simulink model "simulink_discrete1Dy3D_MatLab_function_mascara"  (R2023b)
settings: Solver=ode45  StartTime=0.0  StopTime=0.7  RelTol=1e-3  EnableMultiTasking=on
values from neighbouring files (symbols this model uses):
  a1 = C_discrete.den{1,1}(2)    [control_float_test.m]
  a2 = C_discrete.den{1,1}(3)    [control_float_test.m]
  b0 = C_discrete.num{1,1}(1)    [control_float_test.m]
  b1 = C_discrete.num{1,1}(2)    [control_float_test.m]
  b2 = C_discrete.num{1,1}(3)    [control_float_test.m]
  T = T2    (= 0.001)    [control_float_test.m]
libraries: cstblocks x4
settings Model: Creator=Koldo  LastModifiedBy=chris
settings SolverCC: AlgebraicLoopSolver=TrustRegion
settings DataIOCC: LimitDataPoints=on  SaveFormat=Array  SignalLoggingSaveFormat=ModelDataLogs  ReturnWorkspaceOutputs=off
settings OptimizationCC: ExpressionDepthLimit=2147483647  LifeSpan=inf
settings DebuggingCC: UnderspecifiedInitializationDetection=Classic  MergeDetectMultiDrivingBlocksExec=none  SolverPrmCheckMsg=warning  FcnCallInpInsideContextMsg=warning  UnconnectedInputMsg=warning  UnconnectedOutputMsg=warning  UnconnectedLineMsg=warning  StateNameClashWarn=warning  SFUnexpectedBacktrackingDiag=warning  SFNoUnconditionalDefaultTransitionDiag=warning  SFExecutionAtInitializationDiag=none  ArithmeticOperatorsInVariantConditions=warning
settings HardwareCC: ProdBitPerPointer=32  ProdBitPerSizeT=32  ProdBitPerPtrDiffT=32  ProdLargestAtomicFloat=None  ProdIntDivRoundTo=Undefined  ProdEndianess=Unspecified  ProdWordSize=32  ProdHWDeviceType=32-bit Generic
settings ModelReferenceCC: EnableRefExpFcnMdlSchedulingChecks=on  PropagateSignalLabelsOutOfModel=off
settings SFSimCC: SimUseLocalCustomCode=off  CustomCodeUndefinedFunction=UseInterfaceOnly
settings RTWCC: RTWUseLocalCustomCode=off  DLArmComputeVersion=19.05
settings CodeAppCC: StateflowObjectComments=on
settings GRTTargetCC: TargetLangStandard=C89/C90 (ANSI)  CombineOutputUpdateFcns=off  GRTInterface=on
settings ConfigComp: CovMetricSettings=dw  CovSaveCumulativeToWorkspaceVar=on  CovSaveSingleToWorkspaceVar=on  CovExternalEMLEnable=off

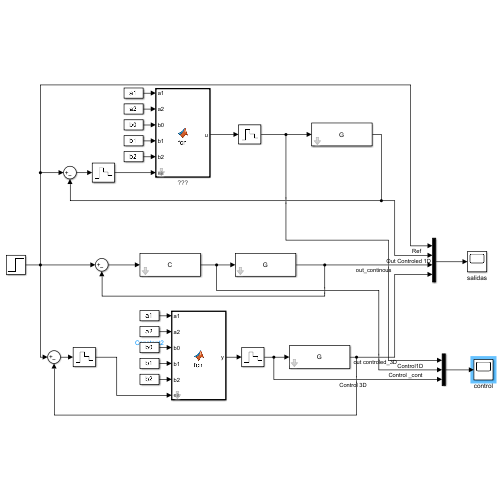
[thumbnail: Simulink's stored preview of the top-level diagram]
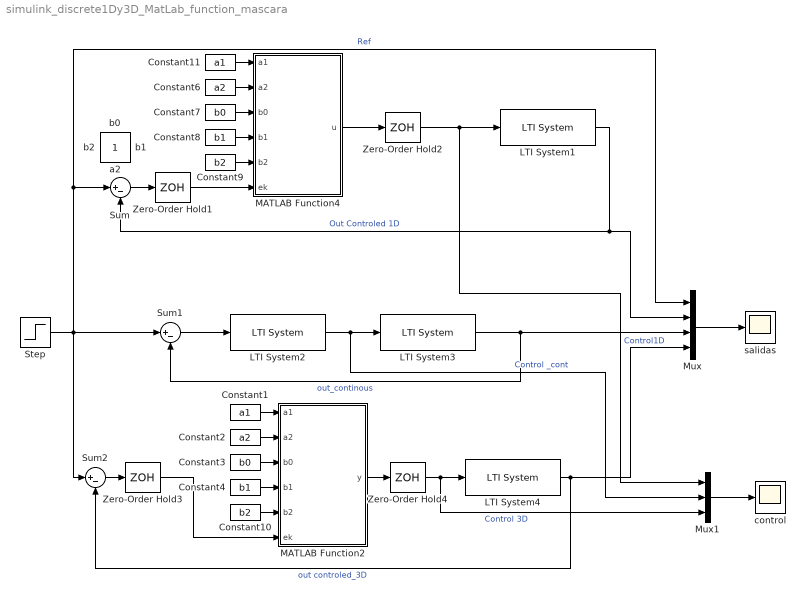
== system simulink_discrete1Dy3D_MatLab_function_mascara ==
  Constant1 : Constant  Value=a1
  Constant10 : Constant  Value=b2
  Constant11 : Constant  Value=a1
  Constant2 : Constant  Value=a2
  Constant3 : Constant  Value=b0
  Constant4 : Constant  Value=b1
  Constant6 : Constant  Value=a2
  Constant7 : Constant  Value=b0
  Constant8 : Constant  Value=b1
  Constant9 : Constant  Value=b2
  LTI System1 : cstblocks/LTI System  sys=G  IC=[]  PadeOrder=0
  LTI System2 : cstblocks/LTI System  sys=C  IC=[]  PadeOrder=0
  LTI System3 : cstblocks/LTI System  sys=G  IC=[]  PadeOrder=0
  LTI System4 : cstblocks/LTI System  sys=G  IC=[]  PadeOrder=0
  MATLAB Function2 : MATLAB Function  TreatAsAtomicUnit=on  mask{a1=0, a2=0, b0=0, b1=0, b2=0}
  MATLAB Function4 : MATLAB Function  TreatAsAtomicUnit=on  mask{Parameter6=double, Parameter7=double, Parameter8=double, Parameter9=double, Parameter10=double}
      mask prompts: Parameter6 "a1"; Parameter7 "a2"; Parameter8 "b0"; Parameter9 "b1"; Parameter10 "b2"
      settings: AttributesFormatString=%<>
  Mux : Mux
  Mux1 : Mux  Inputs=3
  Step : Step  Time=0  After=pi  SampleTime=0
  Sum : Sum  Inputs=|+-
  Sum1 : Sum  Inputs=|+-
  Sum2 : Sum  Inputs=|+-
  Zero-Order Hold{1..4} (4 alike) : ZeroOrderHold  SampleTime=T
  control : Scope
  salidas : Scope
  a2 : Constant  IOType=siggen
  b0 : Constant  IOType=siggen
  b1 : Constant  IOType=siggen
  b2 : Constant  IOType=siggen
  wires:
  Sum/1 -> Zero-Order Hold1/1
  LTI System1/1 -> Mux/2, Sum/2  "Out Controled 1D"
  Zero-Order Hold2/1 -> LTI System1/1, Mux1/1  "Control1D"
  Step/1 -> Sum2/1, Sum1/1, Sum/1, Mux/1  "Ref"
  Sum1/1 -> LTI System2/1
  LTI System3/1 -> Sum1/2, Mux/3  "out_continous"
  LTI System2/1 -> LTI System3/1, Mux1/2  "Control _cont"
  Mux/1 -> salidas/1
  Sum2/1 -> Zero-Order Hold3/1
  LTI System4/1 -> Mux/4, Sum2/2  "out controled_3D"
  Zero-Order Hold3/1 -> MATLAB Function2/6(ek)
  Zero-Order Hold4/1 -> LTI System4/1, Mux1/3  "Control 3D"
  Mux1/1 -> control/1
  MATLAB Function2/1(y) -> Zero-Order Hold4/1
  Zero-Order Hold1/1 -> MATLAB Function4/6(ek)
  MATLAB Function4/1(u) -> Zero-Order Hold2/1
  Constant7/1 -> MATLAB Function4/3(b0)
  Constant11/1 -> MATLAB Function4/1(a1)
  Constant6/1 -> MATLAB Function4/2(a2)
  Constant8/1 -> MATLAB Function4/4(b1)
  Constant9/1 -> MATLAB Function4/5(b2)
  Constant3/1 -> MATLAB Function2/3(b0)
  Constant1/1 -> MATLAB Function2/1(a1)
  Constant2/1 -> MATLAB Function2/2(a2)
  Constant4/1 -> MATLAB Function2/4(b1)
  Constant10/1 -> MATLAB Function2/5(b2)

== matlab function simulink_discrete1Dy3D_MatLab_function_mascara/MATLAB Function4 ==
  data: a1 input; a2 input; b0 input; b1 input; b2 input; u output; ek input
function u = fcn(a1,a2,b0,b1,b2,ek)



    vec= [a1 a2 b0 b1 b2]
    % Registros 1D
    persistent pk1 pk2
    % Forma canónica (2 registros). Sensible a la cuantificación numérica.
    % uk = b0(ek-a1*pk1-a2*pk2) + b1*pk1 + b2*pk2;
    % Inicializamos los registros (reset)
    if isempty (pk1)
        pk1=0;
    end
    if isempty (pk2)
        pk2=0;
    end
    
    %Realimentación
    %ek = setpoints - yk;
    
    %Cálculo de la señal de control
    apk1 = a1*pk1;
    apk2 = a2*pk2;
    pk = ek - apk1 - apk2;
    
    bpk = b0*pk;
    bpk1 = b1*pk1;
    bpk2 = b2*pk2;
    uk = bpk + bpk1 + bpk2;
    
    %Actualizamos los registros
    pk2=pk1;
    pk1=pk;
    u=uk;

== matlab function simulink_discrete1Dy3D_MatLab_function_mascara/MATLAB Function2 ==
  data: a1 input; a2 input; b0 input; b1 input; b2 input; y output; ek input
function y = fcn(a1,a2,b0,b1,b2,ek)
    

    persistent ek1 ek2 uk1 uk2
    % No canónica: cuatro registros
    % u(k) = b0*e(k)+b1*e(k-1)+b2*e(k-2)-a1*u(k-1)-a2*u(k-2)
    if isempty (uk1)
        uk1=0;
     end
     if isempty (uk2)
        uk2=0;
    end
    if isempty (ek1)
        ek1=0;
    end
    if isempty (ek2)
        ek2=0;
    end

    %ek= setpoints-yk;
    uk = b0*ek+b1*ek1+b2*ek2-a1*uk1-a2*uk2;
    uk2=uk1;
    uk1=uk;
    ek2=ek1;
    ek1=ek;
    u =uk;
y = u;
